simulink library "acc"  (R2021b)
settings: Solver=VariableStepAuto  StartTime=0.0  StopTime=10.0  RelTol=1e-3
undefined symbols (not defined in the file or in its folder): AACC_CondensorFanReq_X_enum, AACC_EWP1CCUReq_X_C, AACC_EWP1EDUReq_X_C, AACC_EWP1HVBReq_X_C, AACC_EWP2CCUReq_X_C, AACC_EWP2EDUReq_X_C, AACC_EWP2HVBReq_X_C, AACC_FWV1CCUReq_X_C, AACC_FWV1EDUReq_X_C, AACC_FWV1HVBReq_X_C, AACC_FWV2CCUReq_X_C, AACC_FWV2EDUReq_X_C, AACC_FWV2HVBReq_X_C, AACC_TWVCCUReq_X_C, AACC_TWVEDUReq_X_C, AACC_TWVHVBReq_X_C, ENUM_ACCMODE_CHARGING, ENUM_ACCMODE_COOLING, ENUM_ACCMODE_OFF, ENUM_ACCMODE_SERVICE, ENUM_ACREQ_COOLING, ENUM_ACREQ_NOREQUEST, ENUM_CHILLERINITREQ_NONE, ENUM_CHILLERINITREQ_START, ENUM_CHILLERINITREQ_WAITING, ENUM_CHILLERINITSTA_FINISH, ENUM_CHILLERINITSTA_INPROCESS, ENUM_COOLFANREQ_HI, ENUM_COOLFANREQ_LOW, ENUM_COOLFANREQ_OFF, ENUM_EACENDEM_SHUTDOWN, ENUM_EACENDEM_START, ENUM_EACENSTA_RUN, ENUM_EBSBRKSW_PRESSED, ENUM_EBSBRKSW_RELEASED, ENUM_EHPSENDEM_SHUTDOWN, ENUM_EHPSENDEM_START, ENUM_EPBSTARAW_SET, ENUM_GEARACTUALPOSN_N, ENUM_GEARACTUALPOSN_P, ENUM_LVBATTSTA_FAIL, ENUM_LVBATTSTA_NORMAL, ENUM_PMMMODE_CHARGE, ENUM_PMMMODE_DRIVE, ENUM_PMMMODE_LVBATCHRG, ENUM_PMMMODE_POWERUP, ENUM_POWERSTA_OFF, ENUM_POWERSTA_ON, ENUM_POWERSTA_READY, ENUM_POWERSTA_STANDBY, ENUM_PUSTATE_COMPLETED, ENUM_THCMSYS_INACTIVE, FALSE, KACC_CACEnableFailTime_s, KACC_CCUFanHighOffTemp_C, KACC_CCUFanHighOnTemp_C, KACC_CCUFanLowOffTemp_C, KACC_CCUFanLowOnTemp_C, KACC_ChillerInitTime_s, KACC_ChillerStartTime_s ... (+77)
libraries: hcu_lib x10, simulink x1
(part 2 of 2)

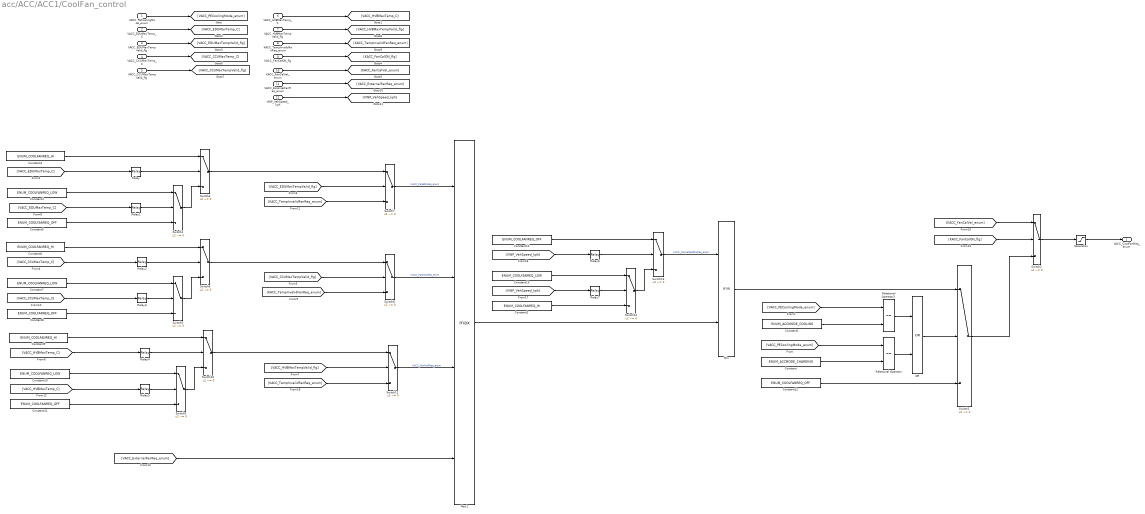
== system acc/ACC/ACC1/CoolFan_control ==
  VACC_PECoolingMode_enum : Inport
  VACC_EDUMaxTemp_C : Inport  Port=2
  VACC_EDUMaxTempValid_flg : Inport  Port=3
  VACC_CCUMaxTemp_C : Inport  Port=4
  VACC_CCUMaxTempValid_flg : Inport  Port=5
  VACC_HVBMaxTemp_C : Inport  Port=6
  VACC_HVBMaxTempValid_flg : Inport  Port=7
  KACC_TempInvalidFanReq_enum : Inport  Port=8
  KACC_FanCalON_flg : Inport  Port=9
  KACC_FanCalVal_enum : Inport  Port=10
  VACC_ExternalFanReq_enum : Inport  Port=11
  VINP_VehSpeed_kph : Inport  Port=12
  Constant : Constant  Value=ENUM_ACCMODE_CHARGING
  Constant1 : Constant  Value=ENUM_ACCMODE_COOLING
  Constant{4,7,10,13} (4 alike) : Constant  Value=ENUM_COOLFANREQ_LOW
  Constant{5,8,11..12,14} (5 alike) : Constant  Value=ENUM_COOLFANREQ_OFF
  Constant{2..3,6,9} (4 alike) : Constant  Value=ENUM_COOLFANREQ_HI
  Max1 : MinMax  Function=max  Inputs=4
  Min : MinMax  Inputs=2
  OR : Logic  Operator=OR  AllPortsSameDT=off  OutDataTypeStr=boolean
  Relational Operator : RelationalOperator  Operator===  OutDataTypeStr=boolean  RndMeth=Simplest
  Relational Operator2 : RelationalOperator  Operator===  OutDataTypeStr=boolean  RndMeth=Simplest
  Relay : Relay  OnSwitchValue=KACC_EDUFanHighOnTemp_C  OffSwitchValue=KACC_EDUFanHighOffTemp_C
      settings: AttributesFormatString=|
      | ON: %<OnSwitchValue>
      | OFF: %<OffSwitchValue>
  Relay1 : Relay  OnSwitchValue=KACC_EDUFanLowOnTemp_C  OffSwitchValue=KACC_EDUFanLowOffTemp_C
      settings: AttributesFormatString=|
      | ON: %<OnSwitchValue>
      | OFF: %<OffSwitchValue>
  Relay2 : Relay  OnSwitchValue=KACC_CCUFanHighOnTemp_C  OffSwitchValue=KACC_CCUFanHighOffTemp_C
      settings: AttributesFormatString=|
      | ON: %<OnSwitchValue>
      | OFF: %<OffSwitchValue>
  Relay3 : Relay  OnSwitchValue=KACC_CCUFanLowOnTemp_C  OffSwitchValue=KACC_CCUFanLowOffTemp_C
      settings: AttributesFormatString=|
      | ON: %<OnSwitchValue>
      | OFF: %<OffSwitchValue>
  Relay4 : Relay  OnSwitchValue=KACC_HVBFanHighOnTemp_C  OffSwitchValue=KACC_HVBFanHighOffTemp_C
      settings: AttributesFormatString=|
      | ON: %<OnSwitchValue>
      | OFF: %<OffSwitchValue>
  Relay5 : Relay  OnSwitchValue=KACC_HVBFanLowOnTemp_C  OffSwitchValue=KACC_HVBFanLowOffTemp_C
      settings: AttributesFormatString=|
      | ON: %<OnSwitchValue>
      | OFF: %<OffSwitchValue>
  Relay6 : Relay  OnSwitchValue=KACC_VehSpdFanLowOff_kph  OffSwitchValue=KACC_VehSpdFanLowOn_kph
      settings: AttributesFormatString=|
      | ON: %<OnSwitchValue>
      | OFF: %<OffSwitchValue>
  Relay7 : Relay  OnSwitchValue=KACC_VehSpdFanHighOff_kph  OffSwitchValue=KACC_VehSpdFanHighOn_kph
      settings: AttributesFormatString=|
      | ON: %<OnSwitchValue>
      | OFF: %<OffSwitchValue>
  Saturation : Saturate  UpperLimit=2  LowerLimit=0
      settings: AttributesFormatString=|
      | LowerLimi: %<LowerLimit>
      | UpperLimit: %<UpperLimit>
  Switch{1..13} (13 alike) : Switch  Criteria=u2 ~= 0
      settings: AttributesFormatString=%<Criteria>
  VACC_CoolFanReq_enum : Outport
  wires:
  Min/1 -> Switch1/1
  Switch13/1 -> Min/1  "VACC_FanVehSpdDisReq_enum"
  Max1/1 -> Min/2
  Constant2/1 -> Switch12/3
  [VINP_VehSpeed_kph] -> Relay7/1
  Constant14/1 -> Switch13/1
  [VINP_VehSpeed_kph] -> Relay6/1
  Switch12/1 -> Switch13/3
  Constant13/1 -> Switch12/1
  Relay7/1 -> Switch12/2
  Relay6/1 -> Switch13/2
  Constant12/1 -> Switch1/3
  [VACC_ExternalFanReq_enum] -> Max1/4
  Switch11/1 -> Max1/3  "VACC_FanHVBReq_enum"
  Switch8/1 -> Max1/2  "VACC_FanCCUReq_enum"
  Switch7/1 -> Max1/1  "VACC_FanEDUReq_enum"
  VINP_VehSpeed_kph/1 -> [VINP_VehSpeed_kph]
  [KACC_TempInvalidFanReq_enum] -> Switch11/3
  Switch10/1 -> Switch11/1
  Constant11/1 -> Switch9/3
  Constant10/1 -> Switch9/1
  Relay5/1 -> Switch9/2
  Switch9/1 -> Switch10/3
  Constant9/1 -> Switch10/1
  Relay4/1 -> Switch10/2
  [VACC_HVBMaxTempValid_flg] -> Switch11/2
  [VACC_HVBMaxTemp_C] -> Relay4/1
  [VACC_HVBMaxTemp_C] -> Relay5/1
  [VACC_CCUMaxTemp_C] -> Relay3/1
  [VACC_CCUMaxTemp_C] -> Relay2/1
  [VACC_CCUMaxTempValid_flg] -> Switch8/2
  Relay2/1 -> Switch6/2
  Constant6/1 -> Switch6/1
  Switch5/1 -> Switch6/3
  Relay3/1 -> Switch5/2
  Constant7/1 -> Switch5/1
  Constant8/1 -> Switch5/3
  Switch6/1 -> Switch8/1
  [KACC_TempInvalidFanReq_enum] -> Switch8/3
  [KACC_TempInvalidFanReq_enum] -> Switch7/3
  [VACC_EDUMaxTempValid_flg] -> Switch7/2
  Switch4/1 -> Switch7/1
  Constant5/1 -> Switch3/3
  Constant4/1 -> Switch3/1
  Relay1/1 -> Switch3/2
  [VACC_EDUMaxTemp_C] -> Relay1/1
  Switch3/1 -> Switch4/3
  Constant3/1 -> Switch4/1
  Relay/1 -> Switch4/2
  [VACC_EDUMaxTemp_C] -> Relay/1
  VACC_ExternalFanReq_enum/1 -> [VACC_ExternalFanReq_enum]
  [KACC_FanCalVal_enum] -> Switch2/1
  [KACC_FanCalON_flg] -> Switch2/2
  KACC_FanCalVal_enum/1 -> [KACC_FanCalVal_enum]
  KACC_FanCalON_flg/1 -> [KACC_FanCalON_flg]
  Saturation/1 -> VACC_CoolFanReq_enum/1
  Switch2/1 -> Saturation/1
  VACC_PECoolingMode_enum/1 -> [VACC_PECoolingMode_enum]
  [VACC_PECoolingMode_enum] -> Relational Operator/1
  [VACC_PECoolingMode_enum] -> Relational Operator2/1
  Constant1/1 -> Relational Operator2/2
  Constant/1 -> Relational Operator/2
  Switch1/1 -> Switch2/3
  VACC_HVBMaxTemp_C/1 -> [VACC_HVBMaxTemp_C]
  Relational Operator2/1 -> OR/1
  Relational Operator/1 -> OR/2
  OR/1 -> Switch1/2
  VACC_EDUMaxTemp_C/1 -> [VACC_EDUMaxTemp_C]
  VACC_EDUMaxTempValid_flg/1 -> [VACC_EDUMaxTempValid_flg]
  VACC_CCUMaxTemp_C/1 -> [VACC_CCUMaxTemp_C]
  VACC_CCUMaxTempValid_flg/1 -> [VACC_CCUMaxTempValid_flg]
  VACC_HVBMaxTempValid_flg/1 -> [VACC_HVBMaxTempValid_flg]
  KACC_TempInvalidFanReq_enum/1 -> [KACC_TempInvalidFanReq_enum]

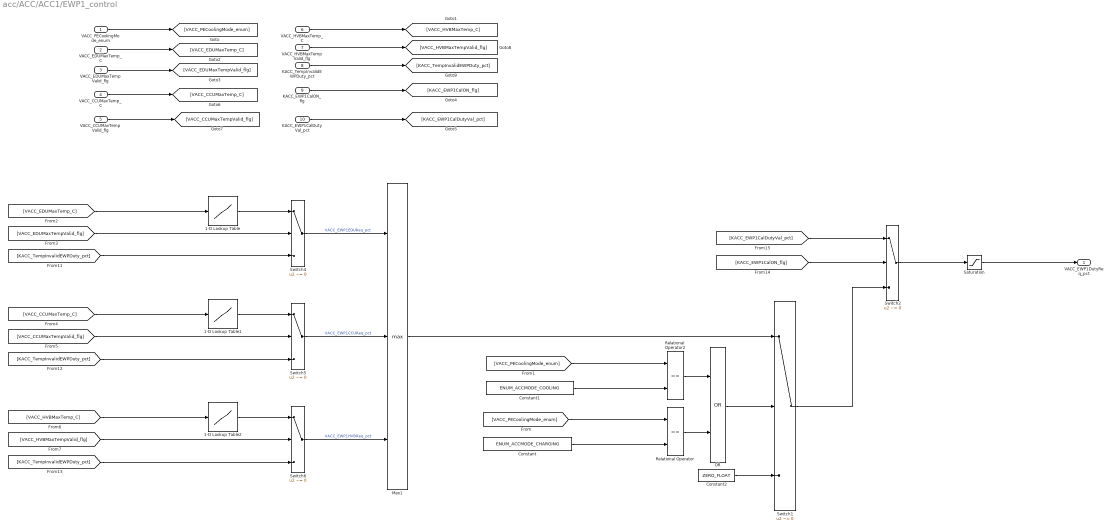
== system acc/ACC/ACC1/EWP1_control ==
  VACC_PECoolingMode_enum : Inport
  VACC_EDUMaxTemp_C : Inport  Port=2
  VACC_EDUMaxTempValid_flg : Inport  Port=3
  VACC_CCUMaxTemp_C : Inport  Port=4
  VACC_CCUMaxTempValid_flg : Inport  Port=5
  VACC_HVBMaxTemp_C : Inport  Port=6
  VACC_HVBMaxTempValid_flg : Inport  Port=7
  KACC_TempInvalidEWPDuty_pct : Inport  Port=8
  KACC_EWP1CalON_flg : Inport  Port=9
  KACC_EWP1CalDutyVal_pct : Inport  Port=10
  1-D Lookup Table : Lookup_n-D  NumberOfTableDimensions=1  BreakpointsForDimension1=AACC_EWP1EDUReq_X_C  Table=MACC_EWP1EDUReq_Y_pct  UseLastTableValue=on  InternalRulePriority=Speed  RndMeth=Simplest  InputSameDT=on
  1-D Lookup Table1 : Lookup_n-D  NumberOfTableDimensions=1  BreakpointsForDimension1=AACC_EWP1CCUReq_X_C  Table=MACC_EWP1CCUReq_Y_pct  UseLastTableValue=on  InternalRulePriority=Speed  RndMeth=Simplest  InputSameDT=on
  1-D Lookup Table2 : Lookup_n-D  NumberOfTableDimensions=1  BreakpointsForDimension1=AACC_EWP1HVBReq_X_C  Table=MACC_EWP1HVBReq_Y_pct  UseLastTableValue=on  InternalRulePriority=Speed  RndMeth=Simplest  InputSameDT=on
  Constant : Constant  Value=ENUM_ACCMODE_CHARGING
  Constant1 : Constant  Value=ENUM_ACCMODE_COOLING
  Constant2 : Constant  Value=ZERO_FLOAT
  Max1 : MinMax  Function=max  Inputs=3
  OR : Logic  Operator=OR  AllPortsSameDT=off  OutDataTypeStr=boolean
  Relational Operator : RelationalOperator  Operator===  OutDataTypeStr=boolean  RndMeth=Simplest
  Relational Operator2 : RelationalOperator  Operator===  OutDataTypeStr=boolean  RndMeth=Simplest
  Saturation : Saturate  UpperLimit=100  LowerLimit=0
      settings: AttributesFormatString=|
      | LowerLimi: %<LowerLimit>
      | UpperLimit: %<UpperLimit>
  Switch{1..2,4..6} (5 alike) : Switch  Criteria=u2 ~= 0
      settings: AttributesFormatString=%<Criteria>
  VACC_EWP1DutyReq_pct : Outport
  wires:
  Saturation/1 -> VACC_EWP1DutyReq_pct/1
  [KACC_EWP1CalDutyVal_pct] -> Switch2/1
  [KACC_EWP1CalON_flg] -> Switch2/2
  [KACC_TempInvalidEWPDuty_pct] -> Switch6/3
  [VACC_HVBMaxTemp_C] -> 1-D Lookup Table2/1
  [VACC_HVBMaxTempValid_flg] -> Switch6/2
  1-D Lookup Table2/1 -> Switch6/1
  Switch6/1 -> Max1/3  "VACC_EWP1HVBReq_pct"
  [KACC_TempInvalidEWPDuty_pct] -> Switch5/3
  [VACC_CCUMaxTempValid_flg] -> Switch5/2
  1-D Lookup Table1/1 -> Switch5/1
  [VACC_CCUMaxTemp_C] -> 1-D Lookup Table1/1
  1-D Lookup Table/1 -> Switch4/1
  [VACC_EDUMaxTemp_C] -> 1-D Lookup Table/1
  [KACC_TempInvalidEWPDuty_pct] -> Switch4/3
  [VACC_EDUMaxTempValid_flg] -> Switch4/2
  KACC_EWP1CalDutyVal_pct/1 -> [KACC_EWP1CalDutyVal_pct]
  KACC_EWP1CalON_flg/1 -> [KACC_EWP1CalON_flg]
  Switch2/1 -> Saturation/1
  VACC_PECoolingMode_enum/1 -> [VACC_PECoolingMode_enum]
  [VACC_PECoolingMode_enum] -> Relational Operator/1
  [VACC_PECoolingMode_enum] -> Relational Operator2/1
  Max1/1 -> Switch1/1
  Constant1/1 -> Relational Operator2/2
  Constant/1 -> Relational Operator/2
  Switch1/1 -> Switch2/3
  VACC_HVBMaxTemp_C/1 -> [VACC_HVBMaxTemp_C]
  Relational Operator2/1 -> OR/1
  Relational Operator/1 -> OR/2
  OR/1 -> Switch1/2
  Constant2/1 -> Switch1/3
  VACC_EDUMaxTemp_C/1 -> [VACC_EDUMaxTemp_C]
  VACC_EDUMaxTempValid_flg/1 -> [VACC_EDUMaxTempValid_flg]
  VACC_CCUMaxTemp_C/1 -> [VACC_CCUMaxTemp_C]
  VACC_CCUMaxTempValid_flg/1 -> [VACC_CCUMaxTempValid_flg]
  VACC_HVBMaxTempValid_flg/1 -> [VACC_HVBMaxTempValid_flg]
  KACC_TempInvalidEWPDuty_pct/1 -> [KACC_TempInvalidEWPDuty_pct]
  Switch4/1 -> Max1/1  "VACC_EWP1EDUReq_pct"
  Switch5/1 -> Max1/2  "VACC_EWP1CCUReq_pct"

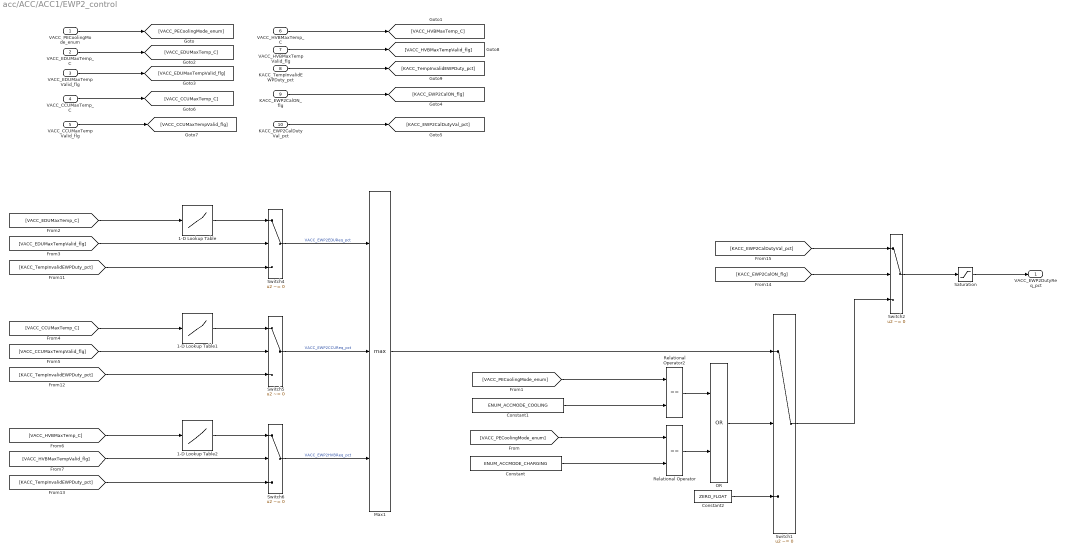
== system acc/ACC/ACC1/EWP2_control ==
  VACC_PECoolingMode_enum : Inport
  VACC_EDUMaxTemp_C : Inport  Port=2
  VACC_EDUMaxTempValid_flg : Inport  Port=3
  VACC_CCUMaxTemp_C : Inport  Port=4
  VACC_CCUMaxTempValid_flg : Inport  Port=5
  VACC_HVBMaxTemp_C : Inport  Port=6
  VACC_HVBMaxTempValid_flg : Inport  Port=7
  KACC_TempInvalidEWPDuty_pct : Inport  Port=8
  KACC_EWP2CalON_flg : Inport  Port=9
  KACC_EWP2CalDutyVal_pct : Inport  Port=10
  1-D Lookup Table : Lookup_n-D  NumberOfTableDimensions=1  BreakpointsForDimension1=AACC_EWP2EDUReq_X_C  Table=MACC_EWP2EDUReq_Y_pct  UseLastTableValue=on  InternalRulePriority=Speed  RndMeth=Simplest  InputSameDT=on
  1-D Lookup Table1 : Lookup_n-D  NumberOfTableDimensions=1  BreakpointsForDimension1=AACC_EWP2CCUReq_X_C  Table=MACC_EWP2CCUReq_Y_pct  UseLastTableValue=on  InternalRulePriority=Speed  RndMeth=Simplest  InputSameDT=on
  1-D Lookup Table2 : Lookup_n-D  NumberOfTableDimensions=1  BreakpointsForDimension1=AACC_EWP2HVBReq_X_C  Table=MACC_EWP2HVBReq_Y_pct  UseLastTableValue=on  InternalRulePriority=Speed  RndMeth=Simplest  InputSameDT=on
  Constant : Constant  Value=ENUM_ACCMODE_CHARGING
  Constant1 : Constant  Value=ENUM_ACCMODE_COOLING
  Constant2 : Constant  Value=ZERO_FLOAT
  Max1 : MinMax  Function=max  Inputs=3
  OR : Logic  Operator=OR  AllPortsSameDT=off  OutDataTypeStr=boolean
  Relational Operator : RelationalOperator  Operator===  OutDataTypeStr=boolean  RndMeth=Simplest
  Relational Operator2 : RelationalOperator  Operator===  OutDataTypeStr=boolean  RndMeth=Simplest
  Saturation : Saturate  UpperLimit=100  LowerLimit=0
      settings: AttributesFormatString=|
      | LowerLimi: %<LowerLimit>
      | UpperLimit: %<UpperLimit>
  Switch{1..2,4..6} (5 alike) : Switch  Criteria=u2 ~= 0
      settings: AttributesFormatString=%<Criteria>
  VACC_EWP2DutyReq_pct : Outport
  wires:
  Switch5/1 -> Max1/2  "VACC_EWP2CCUReq_pct"
  Switch4/1 -> Max1/1  "VACC_EWP2EDUReq_pct"
  KACC_TempInvalidEWPDuty_pct/1 -> [KACC_TempInvalidEWPDuty_pct]
  VACC_HVBMaxTempValid_flg/1 -> [VACC_HVBMaxTempValid_flg]
  VACC_CCUMaxTempValid_flg/1 -> [VACC_CCUMaxTempValid_flg]
  VACC_CCUMaxTemp_C/1 -> [VACC_CCUMaxTemp_C]
  VACC_EDUMaxTempValid_flg/1 -> [VACC_EDUMaxTempValid_flg]
  VACC_EDUMaxTemp_C/1 -> [VACC_EDUMaxTemp_C]
  Constant2/1 -> Switch1/3
  OR/1 -> Switch1/2
  Relational Operator/1 -> OR/2
  Relational Operator2/1 -> OR/1
  VACC_HVBMaxTemp_C/1 -> [VACC_HVBMaxTemp_C]
  Switch1/1 -> Switch2/3
  Constant/1 -> Relational Operator/2
  Constant1/1 -> Relational Operator2/2
  Max1/1 -> Switch1/1
  [VACC_PECoolingMode_enum] -> Relational Operator2/1
  [VACC_PECoolingMode_enum] -> Relational Operator/1
  VACC_PECoolingMode_enum/1 -> [VACC_PECoolingMode_enum]
  Switch2/1 -> Saturation/1
  Saturation/1 -> VACC_EWP2DutyReq_pct/1
  KACC_EWP2CalON_flg/1 -> [KACC_EWP2CalON_flg]
  KACC_EWP2CalDutyVal_pct/1 -> [KACC_EWP2CalDutyVal_pct]
  [VACC_EDUMaxTempValid_flg] -> Switch4/2
  [KACC_TempInvalidEWPDuty_pct] -> Switch4/3
  [VACC_EDUMaxTemp_C] -> 1-D Lookup Table/1
  1-D Lookup Table/1 -> Switch4/1
  [VACC_CCUMaxTemp_C] -> 1-D Lookup Table1/1
  1-D Lookup Table1/1 -> Switch5/1
  [VACC_CCUMaxTempValid_flg] -> Switch5/2
  [KACC_TempInvalidEWPDuty_pct] -> Switch5/3
  Switch6/1 -> Max1/3  "VACC_EWP2HVBReq_pct"
  1-D Lookup Table2/1 -> Switch6/1
  [VACC_HVBMaxTempValid_flg] -> Switch6/2
  [VACC_HVBMaxTemp_C] -> 1-D Lookup Table2/1
  [KACC_TempInvalidEWPDuty_pct] -> Switch6/3
  [KACC_EWP2CalON_flg] -> Switch2/2
  [KACC_EWP2CalDutyVal_pct] -> Switch2/1

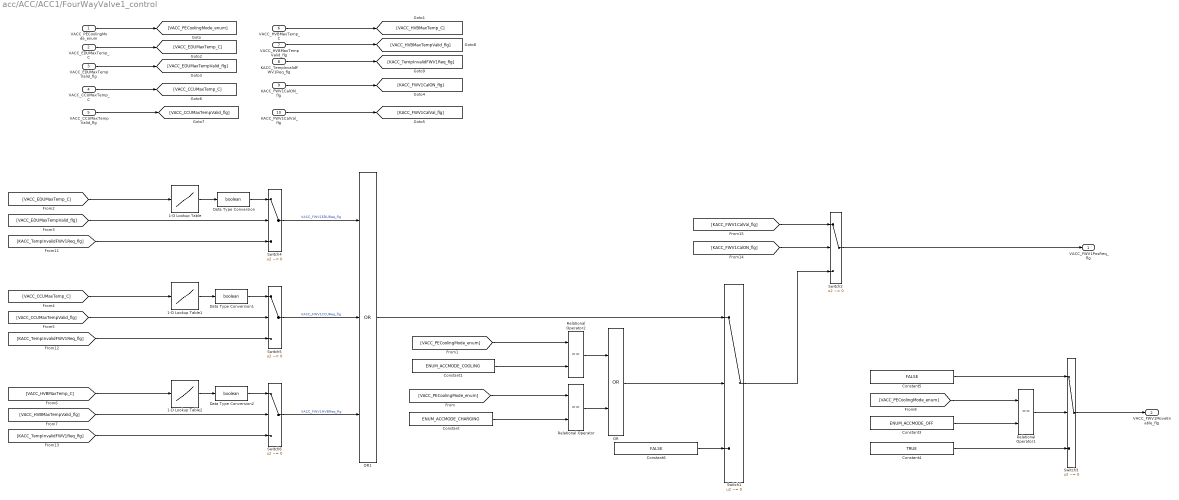
== system acc/ACC/ACC1/FourWayValve1_control ==
  VACC_PECoolingMode_enum : Inport
  VACC_EDUMaxTemp_C : Inport  Port=2
  VACC_EDUMaxTempValid_flg : Inport  Port=3
  VACC_CCUMaxTemp_C : Inport  Port=4
  VACC_CCUMaxTempValid_flg : Inport  Port=5
  VACC_HVBMaxTemp_C : Inport  Port=6
  VACC_HVBMaxTempValid_flg : Inport  Port=7
  KACC_TempInvalidFWV1Req_flg : Inport  Port=8
  KACC_FWV1CalON_flg : Inport  Port=9
  KACC_FWV1CalVal_flg : Inport  Port=10
  1-D Lookup Table : Lookup_n-D  NumberOfTableDimensions=1  BreakpointsForDimension1=AACC_FWV1EDUReq_X_C  Table=MACC_FWV1EDUReq_Y_flg  InterpMethod=Flat  UseLastTableValue=on  InternalRulePriority=Speed  RndMeth=Simplest  InputSameDT=on
  1-D Lookup Table1 : Lookup_n-D  NumberOfTableDimensions=1  BreakpointsForDimension1=AACC_FWV1CCUReq_X_C  Table=MACC_FWV1CCUReq_Y_flg  InterpMethod=Flat  UseLastTableValue=on  InternalRulePriority=Speed  RndMeth=Simplest  InputSameDT=on
  1-D Lookup Table2 : Lookup_n-D  NumberOfTableDimensions=1  BreakpointsForDimension1=AACC_FWV1HVBReq_X_C  Table=MACC_FWV1HVBReq_Y_flg  InterpMethod=Flat  UseLastTableValue=on  InternalRulePriority=Speed  RndMeth=Simplest  InputSameDT=on
  Constant : Constant  Value=ENUM_ACCMODE_CHARGING
  Constant1 : Constant  Value=ENUM_ACCMODE_COOLING
  Constant3 : Constant  Value=ENUM_ACCMODE_OFF
  Constant4 : Constant  Value=TRUE
  Constant5 : Constant  Value=FALSE
  Constant6 : Constant  Value=FALSE
  Data Type Conversion : DataTypeConversion  OutDataTypeStr=boolean
  Data Type Conversion1 : DataTypeConversion  OutDataTypeStr=boolean
  Data Type Conversion2 : DataTypeConversion  OutDataTypeStr=boolean
  OR : Logic  Operator=OR  AllPortsSameDT=off  OutDataTypeStr=boolean
  OR1 : Logic  Operator=OR  Inputs=3  AllPortsSameDT=off  OutDataTypeStr=boolean
  Relational Operator : RelationalOperator  Operator===  OutDataTypeStr=boolean  RndMeth=Simplest
  Relational Operator1 : RelationalOperator  Operator===  OutDataTypeStr=boolean  RndMeth=Simplest
  Relational Operator2 : RelationalOperator  Operator===  OutDataTypeStr=boolean  RndMeth=Simplest
  Switch{1..6} (6 alike) : Switch  Criteria=u2 ~= 0
      settings: AttributesFormatString=%<Criteria>
  VACC_FWV1PosReq_flg : Outport
  VACC_FWV1MoveEnable_flg : Outport  Port=2
  wires:
  Data Type Conversion2/1 -> Switch6/1
  Data Type Conversion1/1 -> Switch5/1
  Data Type Conversion/1 -> Switch4/1
  OR1/1 -> Switch1/1
  Constant6/1 -> Switch1/3
  [KACC_FWV1CalVal_flg] -> Switch2/1
  [KACC_FWV1CalON_flg] -> Switch2/2
  [KACC_TempInvalidFWV1Req_flg] -> Switch6/3
  [VACC_HVBMaxTemp_C] -> 1-D Lookup Table2/1
  [VACC_HVBMaxTempValid_flg] -> Switch6/2
  1-D Lookup Table2/1 -> Data Type Conversion2/1
  Switch6/1 -> OR1/3  "VACC_FWV1HVBReq_flg"
  [KACC_TempInvalidFWV1Req_flg] -> Switch5/3
  [VACC_CCUMaxTempValid_flg] -> Switch5/2
  1-D Lookup Table1/1 -> Data Type Conversion1/1
  [VACC_CCUMaxTemp_C] -> 1-D Lookup Table1/1
  1-D Lookup Table/1 -> Data Type Conversion/1
  [VACC_EDUMaxTemp_C] -> 1-D Lookup Table/1
  [KACC_TempInvalidFWV1Req_flg] -> Switch4/3
  [VACC_EDUMaxTempValid_flg] -> Switch4/2
  KACC_FWV1CalVal_flg/1 -> [KACC_FWV1CalVal_flg]
  KACC_FWV1CalON_flg/1 -> [KACC_FWV1CalON_flg]
  Switch2/1 -> VACC_FWV1PosReq_flg/1
  VACC_PECoolingMode_enum/1 -> [VACC_PECoolingMode_enum]
  [VACC_PECoolingMode_enum] -> Relational Operator/1
  [VACC_PECoolingMode_enum] -> Relational Operator2/1
  Constant1/1 -> Relational Operator2/2
  Constant/1 -> Relational Operator/2
  Switch1/1 -> Switch2/3
  VACC_HVBMaxTemp_C/1 -> [VACC_HVBMaxTemp_C]
  Relational Operator2/1 -> OR/1
  Relational Operator/1 -> OR/2
  OR/1 -> Switch1/2
  VACC_EDUMaxTemp_C/1 -> [VACC_EDUMaxTemp_C]
  VACC_EDUMaxTempValid_flg/1 -> [VACC_EDUMaxTempValid_flg]
  VACC_CCUMaxTemp_C/1 -> [VACC_CCUMaxTemp_C]
  VACC_CCUMaxTempValid_flg/1 -> [VACC_CCUMaxTempValid_flg]
  VACC_HVBMaxTempValid_flg/1 -> [VACC_HVBMaxTempValid_flg]
  KACC_TempInvalidFWV1Req_flg/1 -> [KACC_TempInvalidFWV1Req_flg]
  Switch4/1 -> OR1/1  "VACC_FWV1EDUReq_flg"
  Switch5/1 -> OR1/2  "VACC_FWV1CCUReq_flg"
  Constant3/1 -> Relational Operator1/2
  [VACC_PECoolingMode_enum] -> Relational Operator1/1
  Relational Operator1/1 -> Switch3/2
  Switch3/1 -> VACC_FWV1MoveEnable_flg/1
  Constant5/1 -> Switch3/1
  Constant4/1 -> Switch3/3

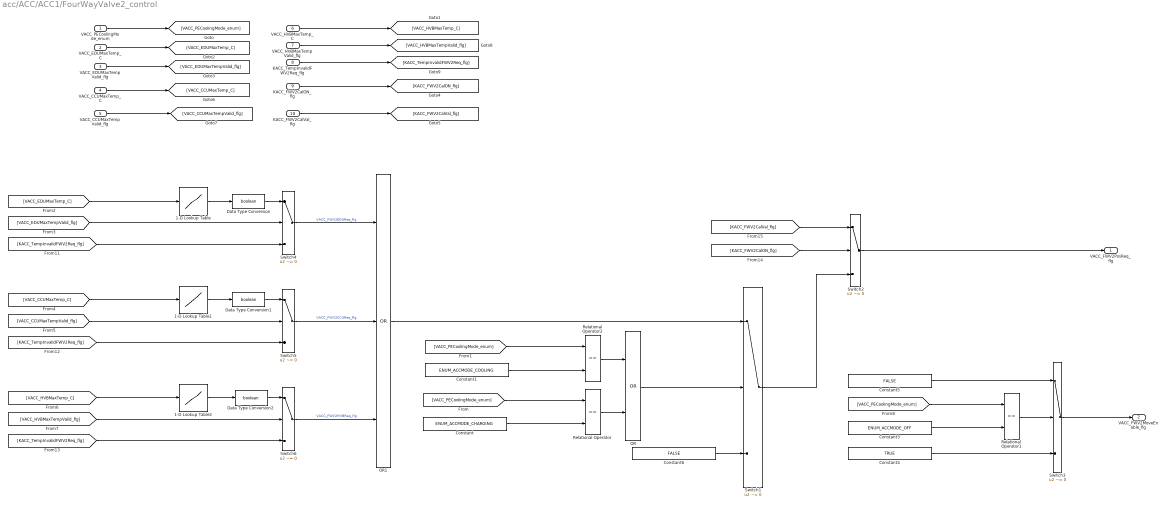
== system acc/ACC/ACC1/FourWayValve2_control ==
  VACC_PECoolingMode_enum : Inport
  VACC_EDUMaxTemp_C : Inport  Port=2
  VACC_EDUMaxTempValid_flg : Inport  Port=3
  VACC_CCUMaxTemp_C : Inport  Port=4
  VACC_CCUMaxTempValid_flg : Inport  Port=5
  VACC_HVBMaxTemp_C : Inport  Port=6
  VACC_HVBMaxTempValid_flg : Inport  Port=7
  KACC_TempInvalidFWV2Req_flg : Inport  Port=8
  KACC_FWV2CalON_flg : Inport  Port=9
  KACC_FWV2CalVal_flg : Inport  Port=10
  1-D Lookup Table : Lookup_n-D  NumberOfTableDimensions=1  BreakpointsForDimension1=AACC_FWV2EDUReq_X_C  Table=MACC_FWV2EDUReq_Y_flg  InterpMethod=Flat  UseLastTableValue=on  InternalRulePriority=Speed  RndMeth=Simplest  InputSameDT=on
  1-D Lookup Table1 : Lookup_n-D  NumberOfTableDimensions=1  BreakpointsForDimension1=AACC_FWV2CCUReq_X_C  Table=MACC_FWV2CCUReq_Y_flg  InterpMethod=Flat  UseLastTableValue=on  InternalRulePriority=Speed  RndMeth=Simplest  InputSameDT=on
  1-D Lookup Table2 : Lookup_n-D  NumberOfTableDimensions=1  BreakpointsForDimension1=AACC_FWV2HVBReq_X_C  Table=MACC_FWV2HVBReq_Y_flg  InterpMethod=Flat  UseLastTableValue=on  InternalRulePriority=Speed  RndMeth=Simplest  InputSameDT=on
  Constant : Constant  Value=ENUM_ACCMODE_CHARGING
  Constant1 : Constant  Value=ENUM_ACCMODE_COOLING
  Constant3 : Constant  Value=ENUM_ACCMODE_OFF
  Constant4 : Constant  Value=TRUE
  Constant5 : Constant  Value=FALSE
  Constant6 : Constant  Value=FALSE
  Data Type Conversion : DataTypeConversion  OutDataTypeStr=boolean
  Data Type Conversion1 : DataTypeConversion  OutDataTypeStr=boolean
  Data Type Conversion2 : DataTypeConversion  OutDataTypeStr=boolean
  OR : Logic  Operator=OR  AllPortsSameDT=off  OutDataTypeStr=boolean
  OR1 : Logic  Operator=OR  Inputs=3  AllPortsSameDT=off  OutDataTypeStr=boolean
  Relational Operator : RelationalOperator  Operator===  OutDataTypeStr=boolean  RndMeth=Simplest
  Relational Operator1 : RelationalOperator  Operator===  OutDataTypeStr=boolean  RndMeth=Simplest
  Relational Operator2 : RelationalOperator  Operator===  OutDataTypeStr=boolean  RndMeth=Simplest
  Switch{1..6} (6 alike) : Switch  Criteria=u2 ~= 0
      settings: AttributesFormatString=%<Criteria>
  VACC_FWV2PosReq_flg : Outport
  VACC_FWV2MoveEnable_flg : Outport  Port=2
  wires:
  Data Type Conversion2/1 -> Switch6/1
  Data Type Conversion1/1 -> Switch5/1
  Data Type Conversion/1 -> Switch4/1
  Constant4/1 -> Switch3/3
  Constant5/1 -> Switch3/1
  Switch3/1 -> VACC_FWV2MoveEnable_flg/1
  Relational Operator1/1 -> Switch3/2
  [VACC_PECoolingMode_enum] -> Relational Operator1/1
  Constant3/1 -> Relational Operator1/2
  Switch5/1 -> OR1/2  "VACC_FWV2CCUReq_flg"
  Switch4/1 -> OR1/1  "VACC_FWV2EDUReq_flg"
  KACC_TempInvalidFWV2Req_flg/1 -> [KACC_TempInvalidFWV2Req_flg]
  VACC_HVBMaxTempValid_flg/1 -> [VACC_HVBMaxTempValid_flg]
  VACC_CCUMaxTempValid_flg/1 -> [VACC_CCUMaxTempValid_flg]
  VACC_CCUMaxTemp_C/1 -> [VACC_CCUMaxTemp_C]
  VACC_EDUMaxTempValid_flg/1 -> [VACC_EDUMaxTempValid_flg]
  VACC_EDUMaxTemp_C/1 -> [VACC_EDUMaxTemp_C]
  OR/1 -> Switch1/2
  Relational Operator/1 -> OR/2
  Relational Operator2/1 -> OR/1
  VACC_HVBMaxTemp_C/1 -> [VACC_HVBMaxTemp_C]
  Switch1/1 -> Switch2/3
  Constant/1 -> Relational Operator/2
  Constant1/1 -> Relational Operator2/2
  [VACC_PECoolingMode_enum] -> Relational Operator2/1
  [VACC_PECoolingMode_enum] -> Relational Operator/1
  VACC_PECoolingMode_enum/1 -> [VACC_PECoolingMode_enum]
  Switch2/1 -> VACC_FWV2PosReq_flg/1
  KACC_FWV2CalON_flg/1 -> [KACC_FWV2CalON_flg]
  KACC_FWV2CalVal_flg/1 -> [KACC_FWV2CalVal_flg]
  [VACC_EDUMaxTempValid_flg] -> Switch4/2
  [KACC_TempInvalidFWV2Req_flg] -> Switch4/3
  [VACC_EDUMaxTemp_C] -> 1-D Lookup Table/1
  1-D Lookup Table/1 -> Data Type Conversion/1
  [VACC_CCUMaxTemp_C] -> 1-D Lookup Table1/1
  1-D Lookup Table1/1 -> Data Type Conversion1/1
  [VACC_CCUMaxTempValid_flg] -> Switch5/2
  [KACC_TempInvalidFWV2Req_flg] -> Switch5/3
  Switch6/1 -> OR1/3  "VACC_FWV2HVBReq_flg"
  1-D Lookup Table2/1 -> Data Type Conversion2/1
  [VACC_HVBMaxTempValid_flg] -> Switch6/2
  [VACC_HVBMaxTemp_C] -> 1-D Lookup Table2/1
  [KACC_TempInvalidFWV2Req_flg] -> Switch6/3
  [KACC_FWV2CalON_flg] -> Switch2/2
  [KACC_FWV2CalVal_flg] -> Switch2/1
  Constant6/1 -> Switch1/3
  OR1/1 -> Switch1/1

== system acc/ACC/ACC1/Signal_convert ==
  VINP_MCUTemp_C : Inport
  VINP_MCUTempValid_flg : Inport  Port=2
  VINP_TMTemp_C : Inport  Port=3
  VINP_TMTempValid_flg : Inport  Port=4
  VINP_DCDCTemp_C : Inport  Port=5
  VINP_DCDCTempValid_flg : Inport  Port=6
  VINP_OBCTemp_C : Inport  Port=7
  VINP_OBCTempValid_flg : Inport  Port=8
  VINP_HVBMTempMax_C : Inport  Port=9
  VINP_HVBMTempMaxValid_flg : Inport  Port=10
  VINP_CondensorFanReq_enum : Inport  Port=11
  1-D Lookup Table : Lookup_n-D  NumberOfTableDimensions=1  BreakpointsForDimension1=AACC_CondensorFanReq_X_enum  Table=MACC_CondensorFanReq_Y_enum  InterpMethod=Flat  InternalRulePriority=Speed  RndMeth=Simplest  InputSameDT=on
  Data Type Conversion : DataTypeConversion  OutDataTypeStr=single
  Data Type Conversion1 : DataTypeConversion  OutDataTypeStr=boolean
  Max2 : MinMax  Function=max  Inputs=2
  Max3 : MinMax  Function=max  Inputs=2
  OR2 : Logic  AllPortsSameDT=off  OutDataTypeStr=boolean
  OR3 : Logic  AllPortsSameDT=off  OutDataTypeStr=boolean
  VACC_EDUMaxTemp_C : Outport
  VACC_EDUMaxTempValid_flg : Outport  Port=2
  VACC_CCUMaxTemp_C : Outport  Port=3
  VACC_CCUMaxTempValid_flg : Outport  Port=4
  VACC_HVBMaxTemp_C : Outport  Port=5
  VACC_HVBMaxTempValid_flg : Outport  Port=6
  VACC_ExternalFanReq_enum : Outport  Port=7
  wires:
  Data Type Conversion1/1 -> VACC_HVBMaxTempValid_flg/1
  Data Type Conversion/1 -> VACC_HVBMaxTemp_C/1
  1-D Lookup Table/1 -> VACC_ExternalFanReq_enum/1
  VINP_CondensorFanReq_enum/1 -> 1-D Lookup Table/1
  VINP_HVBMTempMaxValid_flg/1 -> Data Type Conversion1/1
  VINP_HVBMTempMax_C/1 -> Data Type Conversion/1
  OR3/1 -> VACC_CCUMaxTempValid_flg/1
  Max3/1 -> VACC_CCUMaxTemp_C/1
  VINP_OBCTempValid_flg/1 -> OR3/2
  VINP_DCDCTempValid_flg/1 -> OR3/1
  VINP_DCDCTemp_C/1 -> Max3/1
  VINP_OBCTemp_C/1 -> Max3/2
  OR2/1 -> VACC_EDUMaxTempValid_flg/1
  VINP_TMTempValid_flg/1 -> OR2/2
  VINP_MCUTempValid_flg/1 -> OR2/1
  Max2/1 -> VACC_EDUMaxTemp_C/1
  VINP_TMTemp_C/1 -> Max2/2
  VINP_MCUTemp_C/1 -> Max2/1

== system acc/ACC/ACC1/Thermal_Managemant_Mode_Determination ==
  VPMM_SysPowerMode_enum : Inport
  Constant : Constant  Value=KACC_ServiceModeON_flg
  Cooling Mode : Subsystem
  PECoolingMode : Subsystem
  Service Mode : Subsystem
  Subsystem : Subsystem
  VACC_PECoolingMode_enum : Outport  VectorParamsAs1DForOutWhenUnconnected=off
  wires:
  Constant/1 -> Service Mode/1(KACC_ServiceModeON_flg)
  [VACC_CoolingMode_flg] -> PECoolingMode/3(VACC_CoolingMode_flg)
  [VACC_ChargingMode_flg] -> PECoolingMode/2(VACC_ChargingMode_flg)
  [VACC_ServiceMode_flg] -> PECoolingMode/1(VACC_ServiceMode_flg)
  [VPMM_SysPowerMode_enum] -> Subsystem/1(VPMM_SysPowerMode_enum)
  Subsystem/1(VACC_CoolingMode_flg) -> [VACC_CoolingMode_flg]
  PECoolingMode/1(VACC_PECoolingMode_enum) -> VACC_PECoolingMode_enum/1
  [VPMM_SysPowerMode_enum] -> Cooling Mode/1(VPMM_SysPowerMode_enum)
  VPMM_SysPowerMode_enum/1 -> [VPMM_SysPowerMode_enum]
  Service Mode/1(VACC_ServiceMode_flg) -> [VACC_ServiceMode_flg]
  Cooling Mode/1(VACC_ChargingMode_flg) -> [VACC_ChargingMode_flg]

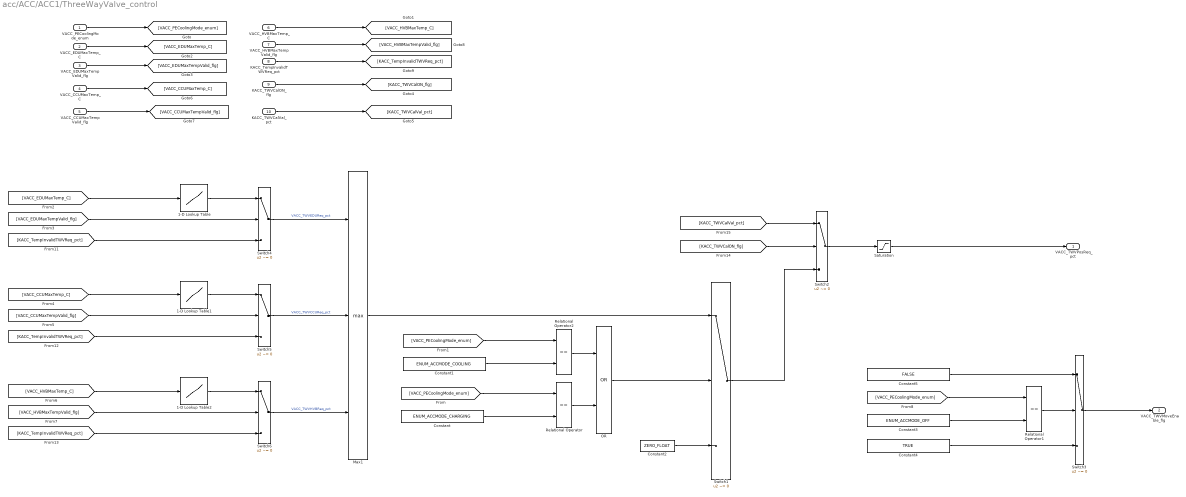
== system acc/ACC/ACC1/ThreeWayValve_control ==
  VACC_PECoolingMode_enum : Inport
  VACC_EDUMaxTemp_C : Inport  Port=2
  VACC_EDUMaxTempValid_flg : Inport  Port=3
  VACC_CCUMaxTemp_C : Inport  Port=4
  VACC_CCUMaxTempValid_flg : Inport  Port=5
  VACC_HVBMaxTemp_C : Inport  Port=6
  VACC_HVBMaxTempValid_flg : Inport  Port=7
  KACC_TempInvalidTWVReq_pct : Inport  Port=8
  KACC_TWVCalON_flg : Inport  Port=9
  KACC_TWVCalVal_pct : Inport  Port=10
  1-D Lookup Table : Lookup_n-D  NumberOfTableDimensions=1  BreakpointsForDimension1=AACC_TWVEDUReq_X_C  Table=MACC_TWVEDUReq_Y_pct  UseLastTableValue=on  InternalRulePriority=Speed  RndMeth=Simplest  InputSameDT=on
  1-D Lookup Table1 : Lookup_n-D  NumberOfTableDimensions=1  BreakpointsForDimension1=AACC_TWVCCUReq_X_C  Table=MACC_TWVCCUReq_Y_pct  UseLastTableValue=on  InternalRulePriority=Speed  RndMeth=Simplest  InputSameDT=on
  1-D Lookup Table2 : Lookup_n-D  NumberOfTableDimensions=1  BreakpointsForDimension1=AACC_TWVHVBReq_X_C  Table=MACC_TWVHVBReq_Y_pct  UseLastTableValue=on  InternalRulePriority=Speed  RndMeth=Simplest  InputSameDT=on
  Constant : Constant  Value=ENUM_ACCMODE_CHARGING
  Constant1 : Constant  Value=ENUM_ACCMODE_COOLING
  Constant2 : Constant  Value=ZERO_FLOAT
  Constant3 : Constant  Value=ENUM_ACCMODE_OFF
  Constant4 : Constant  Value=TRUE
  Constant5 : Constant  Value=FALSE
  Max1 : MinMax  Function=max  Inputs=3
  OR : Logic  Operator=OR  AllPortsSameDT=off  OutDataTypeStr=boolean
  Relational Operator : RelationalOperator  Operator===  OutDataTypeStr=boolean  RndMeth=Simplest
  Relational Operator1 : RelationalOperator  Operator===  OutDataTypeStr=boolean  RndMeth=Simplest
  Relational Operator2 : RelationalOperator  Operator===  OutDataTypeStr=boolean  RndMeth=Simplest
  Saturation : Saturate  UpperLimit=100  LowerLimit=0
      settings: AttributesFormatString=|
      | LowerLimi: %<LowerLimit>
      | UpperLimit: %<UpperLimit>
  Switch{1..6} (6 alike) : Switch  Criteria=u2 ~= 0
      settings: AttributesFormatString=%<Criteria>
  VACC_TWVPosReq_pct : Outport
  VACC_TWVMoveEnable_flg : Outport  Port=2
  wires:
  Constant4/1 -> Switch3/3
  Constant5/1 -> Switch3/1
  Switch3/1 -> VACC_TWVMoveEnable_flg/1
  Relational Operator1/1 -> Switch3/2
  [VACC_PECoolingMode_enum] -> Relational Operator1/1
  Constant3/1 -> Relational Operator1/2
  Switch5/1 -> Max1/2  "VACC_TWVCCUReq_pct"
  Switch4/1 -> Max1/1  "VACC_TWVEDUReq_pct"
  KACC_TempInvalidTWVReq_pct/1 -> [KACC_TempInvalidTWVReq_pct]
  VACC_HVBMaxTempValid_flg/1 -> [VACC_HVBMaxTempValid_flg]
  VACC_CCUMaxTempValid_flg/1 -> [VACC_CCUMaxTempValid_flg]
  VACC_CCUMaxTemp_C/1 -> [VACC_CCUMaxTemp_C]
  VACC_EDUMaxTempValid_flg/1 -> [VACC_EDUMaxTempValid_flg]
  VACC_EDUMaxTemp_C/1 -> [VACC_EDUMaxTemp_C]
  Constant2/1 -> Switch1/3
  OR/1 -> Switch1/2
  Relational Operator/1 -> OR/2
  Relational Operator2/1 -> OR/1
  VACC_HVBMaxTemp_C/1 -> [VACC_HVBMaxTemp_C]
  Switch1/1 -> Switch2/3
  Constant/1 -> Relational Operator/2
  Constant1/1 -> Relational Operator2/2
  Max1/1 -> Switch1/1
  [VACC_PECoolingMode_enum] -> Relational Operator2/1
  [VACC_PECoolingMode_enum] -> Relational Operator/1
  VACC_PECoolingMode_enum/1 -> [VACC_PECoolingMode_enum]
  Switch2/1 -> Saturation/1
  Saturation/1 -> VACC_TWVPosReq_pct/1
  KACC_TWVCalON_flg/1 -> [KACC_TWVCalON_flg]
  KACC_TWVCalVal_pct/1 -> [KACC_TWVCalVal_pct]
  [VACC_EDUMaxTempValid_flg] -> Switch4/2
  [KACC_TempInvalidTWVReq_pct] -> Switch4/3
  [VACC_EDUMaxTemp_C] -> 1-D Lookup Table/1
  1-D Lookup Table/1 -> Switch4/1
  [VACC_CCUMaxTemp_C] -> 1-D Lookup Table1/1
  1-D Lookup Table1/1 -> Switch5/1
  [VACC_CCUMaxTempValid_flg] -> Switch5/2
  [KACC_TempInvalidTWVReq_pct] -> Switch5/3
  Switch6/1 -> Max1/3  "VACC_TWVHVBReq_pct"
  1-D Lookup Table2/1 -> Switch6/1
  [VACC_HVBMaxTempValid_flg] -> Switch6/2
  [VACC_HVBMaxTemp_C] -> 1-D Lookup Table2/1
  [KACC_TempInvalidTWVReq_pct] -> Switch6/3
  [KACC_TWVCalON_flg] -> Switch2/2
  [KACC_TWVCalVal_pct] -> Switch2/1

== system acc/ACC/ACC1/Thermal_Managemant_Mode_Determination/Cooling Mode ==
  VPMM_SysPowerMode_enum : Inport
  Constant2 : Constant  Value=ENUM_PMMMODE_LVBATCHRG  SampleTime=-1
  Constant4 : Constant  Value=ENUM_PMMMODE_CHARGE  SampleTime=-1
  Logical Operator : Logic  Operator=OR  AllPortsSameDT=off  OutDataTypeStr=boolean
  Relational Operator1 : RelationalOperator  Operator===  OutDataTypeStr=boolean  RndMeth=Nearest
  Relational Operator3 : RelationalOperator  Operator===  OutDataTypeStr=boolean  RndMeth=Nearest
  VACC_ChargingMode_flg : Outport  VectorParamsAs1DForOutWhenUnconnected=off
  wires:
  [VPMM_SysPowerMode_enum] -> Relational Operator3/1
  Constant2/1 -> Relational Operator3/2
  VPMM_SysPowerMode_enum/1 -> [VPMM_SysPowerMode_enum]
  [VPMM_SysPowerMode_enum] -> Relational Operator1/1
  Constant4/1 -> Relational Operator1/2
  Relational Operator3/1 -> Logical Operator/1
  Relational Operator1/1 -> Logical Operator/2
  Logical Operator/1 -> VACC_ChargingMode_flg/1  "VACC_ChargingMode_flg"

== system acc/ACC/ACC1/Thermal_Managemant_Mode_Determination/PECoolingMode ==
  VACC_ServiceMode_flg : Inport
  VACC_ChargingMode_flg : Inport  Port=2
  VACC_CoolingMode_flg : Inport  Port=3
  Constant12 : Constant  Value=ENUM_ACCMODE_COOLING  SampleTime=-1
  Constant15 : Constant  Value=ENUM_ACCMODE_OFF  SampleTime=-1
  Constant2 : Constant  Value=ENUM_ACCMODE_CHARGING  SampleTime=-1
  Constant7 : Constant  Value=ENUM_ACCMODE_SERVICE  SampleTime=-1
  Switch1 : Switch  Criteria=u2 ~= 0
  Switch2 : Switch  Criteria=u2 ~= 0
  Switch4 : Switch  Criteria=u2 ~= 0
  VACC_PECoolingMode_enum : Outport  VectorParamsAs1DForOutWhenUnconnected=off
  wires:
  Constant15/1 -> Switch1/3
  Switch4/1 -> VACC_PECoolingMode_enum/1  "VACC_PECoolingMode_enum"
  VACC_CoolingMode_flg/1 -> Switch1/2
  Constant12/1 -> Switch1/1
  VACC_ServiceMode_flg/1 -> Switch4/2
  Constant7/1 -> Switch4/1
  Switch2/1 -> Switch4/3
  VACC_ChargingMode_flg/1 -> Switch2/2
  Switch1/1 -> Switch2/3
  Constant2/1 -> Switch2/1

== system acc/ACC/ACC1/Thermal_Managemant_Mode_Determination/Service Mode ==
  KACC_ServiceModeON_flg : Inport
  VACC_ServiceMode_flg : Outport  VectorParamsAs1DForOutWhenUnconnected=off
  wires:
  KACC_ServiceModeON_flg/1 -> VACC_ServiceMode_flg/1  "VACC_ServiceMode_flg"

== system acc/ACC/ACC1/Thermal_Managemant_Mode_Determination/Subsystem ==
  VPMM_SysPowerMode_enum : Inport
  Constant1 : Constant  Value=ENUM_PMMMODE_DRIVE  SampleTime=-1
  Constant2 : Constant  Value=ENUM_PMMMODE_POWERUP  SampleTime=-1
  Logical Operator : Logic  Operator=OR  AllPortsSameDT=off  OutDataTypeStr=boolean
  Relational Operator1 : RelationalOperator  Operator===  OutDataTypeStr=boolean  RndMeth=Nearest
  Relational Operator2 : RelationalOperator  Operator===  OutDataTypeStr=boolean  RndMeth=Nearest
  VACC_CoolingMode_flg : Outport  VectorParamsAs1DForOutWhenUnconnected=off
  wires:
  Logical Operator/1 -> VACC_CoolingMode_flg/1  "VACC_CoolingMode_flg"
  Relational Operator1/1 -> Logical Operator/2
  Relational Operator2/1 -> Logical Operator/1
  VPMM_SysPowerMode_enum/1 -> [VPMM_SysPowerMode_enum]
  [VPMM_SysPowerMode_enum] -> Relational Operator2/1
  [VPMM_SysPowerMode_enum] -> Relational Operator1/1
  Constant1/1 -> Relational Operator1/2
  Constant2/1 -> Relational Operator2/2

== stateflow chart acc/ACC/ACC/LVBattSta_Check ==
  state Check_LV_Batt
    state Check_LVBatt_Low
      en:
      VACC_ChkLVBattLowPass_flg = FALSE;
      (default) -> (junction 148) : {VACC_LVBattChkTime_s = 0;}
      (junction 148) -> (junction 149) [order 1] : [VINP_LVBattDet12V_V > KACC_LVBattErrLoThd_V]
      Check_LVBatt_Low -> (junction 148) [order 1]
      (junction 148) -> (junction 150) [order 2] : {VACC_LVBattChkTime_s += task_time_s;}
      (junction 149) -> (junction 151) : {VACC_ChkLVBattLowPass_flg = TRUE;}
      (junction 151) -> (junction 150)
    state Check_LVBatt_High
      en:
      VACC_ChkLVBattHighPass_flg = FALSE;
      (default) -> (junction 159) : {VACC_LVBattChkTime_s = 0;}
      Check_LVBatt_High -> (junction 159) [order 1]
      (junction 159) -> (junction 160) [order 1] : [VINP_LVBattDet12V_V < KACC_LVBattErrHiThd_V]
      (junction 159) -> (junction 161) [order 2] : {VACC_LVBattChkTime_s += task_time_s;}
      (junction 160) -> (junction 162) : {VACC_ChkLVBattHighPass_flg = TRUE;}
      (junction 162) -> (junction 161)
    state Check_LVBatt_Pass
      en:
      VACC_LVBattVoltSta_enum = ENUM_LVBATTSTA_NORMAL;
    state Check_LVBatt_Fail
      en:
      VACC_LVBattVoltSta_enum = ENUM_LVBATTSTA_FAIL;
    (default) -> (junction 130)
    (junction 182) -> (junction 130)
    (junction 180) -> (junction 182)
    (junction 130) -> (junction 132)
    (junction 132) -> (junction 131) [order 2]
    (junction 131) -> Check_LVBatt_Pass
    (junction 132) -> Check_LVBatt_Low [order 1] : [VPMM_LVPwrSta_flg]
    Check_LVBatt_Low -> (junction 133) [order 2] : [VACC_LVBattChkTime_s > KACC_LVBattErrFailtime_s]
    (junction 133) -> (junction 134)
    Check_LVBatt_Low -> Check_LVBatt_High [order 1] : [VACC_ChkLVBattLowPass_flg]
    Check_LVBatt_High -> (junction 134) [order 2] : [VACC_LVBattChkTime_s > KACC_LVBattErrFailtime_s]
    (junction 134) -> Check_LVBatt_Fail
    Check_LVBatt_High -> Check_LVBatt_Pass [order 1] : [VACC_ChkLVBattHighPass_flg]
    Check_LVBatt_Pass -> (junction 173)
    Check_LVBatt_Fail -> (junction 175)
    (junction 173) -> (junction 180)
    (junction 175) -> (junction 173)
  data: task_time_s input; VPMM_LVPwrSta_flg input; VINP_LVBattDet12V_V input; KACC_LVBattErrLoThd_V input; KACC_LVBattErrHiThd_V input; KACC_LVBattErrFailtime_s input; VACC_LVBattVoltSta_enum output uint8; VACC_ChkLVBattHighPass_flg local boolean; VACC_ChkLVBattLowPass_flg local boolean; VACC_LVBattChkTime_s local single; ENUM_LVBATTSTA_FAIL parameter; ENUM_LVBATTSTA_NORMAL parameter; FALSE parameter; TRUE parameter

== stateflow chart acc/ACC/ACC/EAC ==
  state EAC_Step_1
    VACC_EACPreSelfChkSta_flg = FALSE;
    state EAC_Enable
      (default) -> (junction 9) : {VACC_TimeEnSta_s = 0;
          |  VACC_EACEnDone_flg = FALSE;}
      (junction 9) -> (junction 14) [order 1] : [VINP_EACEnSta_enum == ENUM_EACENSTA_RUN]
      EAC_Enable -> (junction 9) [order 1]
      (junction 9) -> (junction 12) [order 2] : {VACC_TimeEnSta_s += task_time;}
      (junction 14) -> (junction 16) : {VACC_EACEnDone_flg = TRUE;}
      (junction 16) -> (junction 12)
    state TempStation
    (default) -> (junction 2) : {VACC_EACStep1Done_flg = FALSE;
        |  VACC_EACStep1Loop_flg = TRUE;}
    (junction 2) -> (junction 6) [order 2]
    (junction 2) -> EAC_Enable [order 1] : [VPMM_PowerSta_enum == ENUM_POWERSTA_ON]
        | {VACC_FEACEnDemand_enum = ENUM_EACENDEM_START;
        |  VACC_EACStep1Loop_flg = FALSE;}
        | %add20240718
    (junction 6) -> TempStation : {VACC_EACStep1Done_flg = FALSE;
        |  VACC_EACStep1Loop_flg = TRUE;}
    EAC_Enable -> (junction 21) [order 2] : [VACC_TimeEnSta_s > KACC_CACEnableFailTime_s]
    (junction 21) -> (junction 27) : {VACC_CACPresWarnSta_flg = TRUE;
        |  VACC_FEACEnDemand_enum = ENUM_EACENDEM_SHUTDOWN;}
    EAC_Enable -> (junction 25) [order 1] : [VACC_EACEnDone_flg]
    (junction 27) -> (junction 25)
    (junction 25) -> TempStation : {VACC_EACStep1Done_flg = TRUE;}
  state EAC_Step_2
    ex: VACC_EACPreSelfChkSta_flg = FALSE;
    (default) -> (junction 40)
    EAC_Step_2 -> (junction 40) [order 2]
    (junction 40) -> (junction 42) [order 1] : [VINP_Z24CHAAirPressureRC1Sta_kPa < 700 ||...
        |  VINP_Z24CHAAirPressureFC2Sta_kPa < 700 ||...
        |  VINP_Z24CHAAirPressurePC3Sta_kPa < 700]
    (junction 40) -> (junction 46) [order 2]
    (junction 42) -> (junction 44) : {VACC_CACPresWarnSta_flg = TRUE;}
    (junction 44) -> (junction 46)
    (junction 46) -> (junction 49)
    (junction 49) -> (junction 52) [order 1] : [VINP_Z24CHAAirPressureRC1Sta_kPa < 800 ||...
        |  VINP_Z24CHAAirPressureFC2Sta_kPa < 800]
    (junction 49) -> (junction 70) [order 2]
    (junction 52) -> (junction 150) : {VACC_FEACEnDemand_enum = ENUM_EACENDEM_START;
        |  VACC_TimeEnSta_s = 0;
        |  VACC_EACEnLoop_flg = TRUE;}
    EAC_Step_2 -> (junction 150) [order 1] : [VACC_EACEnLoop_flg]
    (junction 150) -> (junction 155) [order 2]
    (junction 155) -> (junction 73) [order 1] : [VACC_TimeEnSta_s > KACC_CACEnableFailTime_s]
    (junction 150) -> (junction 69) [order 1] : [VINP_EACEnSta_enum == ENUM_EACENSTA_RUN]
        | {VACC_EACEnLoop_flg = FALSE;}
    (junction 155) -> (junction 157) [order 2] : {VACC_TimeEnSta_s += task_time;}
    (junction 73) -> (junction 159) : {VACC_CACPresWarnSta_flg = TRUE;
        |  VACC_FEACEnDemand_enum = ENUM_EACENDEM_SHUTDOWN;
        |  VACC_EACEnLoop_flg = FALSE;}
    (junction 69) -> (junction 70)
    (junction 157) -> (junction 159)
    (junction 70) -> (junction 76)
    (junction 159) -> (junction 162)
    (junction 76) -> (junction 78) [order 1] : [VINP_Z24CHAAirPressureRC1Sta_kPa > 800 &&...
        |  VINP_Z24CHAAirPressureFC2Sta_kPa > 800]
    (junction 76) -> (junction 82) [order 2]
    (junction 78) -> (junction 80) : {VACC_EACPreSelfChkSta_flg = TRUE;}
    (junction 80) -> (junction 82)
    (junction 82) -> (junction 85)
    (junction 85) -> (junction 87) [order 1] : [VINP_Z24CHAAirPressureRC1Sta_kPa > 950 &&...
        |  VINP_Z24CHAAirPressureFC2Sta_kPa > 950]
    (junction 87) -> (junction 91) [order 1] : [VACC_TimePresEnough_s > KACC_TimePresEnoughThd_s]
    (junction 85) -> (junction 96) [order 2] : {VACC_TimePresEnough_s = 0;}
    (junction 87) -> (junction 89) [order 2] : {VACC_TimePresEnough_s += task_time;}
    (junction 91) -> (junction 93) : {VACC_CACPresWarnSta_flg = FALSE;
        |  VACC_CACTempWarnSta_flg = FALSE;
        |  VACC_FEACEnDemand_enum = ENUM_EACENDEM_SHUTDOWN;}
    (junction 89) -> (junction 93)
    (junction 93) -> (junction 113)
    (junction 96) -> (junction 98) [order 1] : [VACC_FEACEnDemand_enum == ENUM_EACENDEM_START]
    (junction 98) -> (junction 102) [order 1] : [VACC_TimeEACEnDem_s > KACC_TimeEACEnDemThd_s]
    (junction 96) -> (junction 106) [order 2] : {VACC_TimeEACEnDem_s = 0;}
    (junction 98) -> (junction 100) [order 2] : {VACC_TimeEACEnDem_s += task_time;}
    (junction 102) -> (junction 104) : {VACC_CACTempWarnSta_flg = TRUE;}
    (junction 100) -> (junction 104)
    (junction 104) -> (junction 148)
  (default) -> EAC_Step_1
  EAC_Step_1 -> EAC_Step_1 [order 2] : [VACC_EACStep1Loop_flg]
  EAC_Step_1 -> EAC_Step_2 [order 1] : [VACC_EACStep1Done_flg]
  EAC_Step_2 -> EAC_Step_1 [order 1] : [VPMM_PowerSta_enum == ENUM_POWERSTA_OFF ||...
      |  VPMM_PowerSta_enum == ENUM_POWERSTA_STANDBY]
  data: VPMM_PowerUpState_enum input; KACC_CACEnableFailTime_s parameter; KACC_TimeEACEnDemThd_s parameter; KACC_TimePresEnoughThd_s parameter; VINP_EACEnSta_enum input; VINP_Z24CHAAirPressureFC2Sta_kPa input; VINP_Z24CHAAirPressurePC3Sta_kPa input; VINP_Z24CHAAirPressureRC1Sta_kPa input; task_time input; VACC_CACPresWarnSta_flg output boolean; VACC_CACTempWarnSta_flg output boolean; VACC_EACPreSelfChkSta_flg output boolean; VACC_EACEnDone_flg local boolean; VACC_EACStep1Done_flg local boolean; VACC_FEACEnDemand_enum output uint8; VACC_TimeEACEnDem_s local single; VACC_TimeEnSta_s local single; VACC_TimePresEnough_s local single; ENUM_EACENDEM_SHUTDOWN parameter; ENUM_EACENDEM_START parameter; ENUM_EACENSTA_RUN parameter; ENUM_PUSTATE_COMPLETED parameter; FALSE parameter; TRUE parameter; VPMM_PowerSta_enum input; ENUM_POWERSTA_OFF parameter; ENUM_POWERSTA_STANDBY parameter; VACC_EACEnLoop_flg local boolean; VACC_EACStep1Loop_flg local boolean; ENUM_POWERSTA_ON parameter

== stateflow chart acc/ACC/ACC1/Chiller_control/Chiller_Initialize ==
  state MainInitialize
    en:
    VACC_ChillerInitFinish_flg = FALSE;
    VACC_ChillerInitTimeout_flg = FALSE;
    VACC_ChillerInitStart_flg = FALSE;
    VACC_ChillerInitReq_enum = ENUM_CHILLERINITREQ_NONE;
    VACC_ChillerMoveEnable_flg = FALSE;
  state ChillerInitialize
    (default) -> (junction 10) : {
        | VACC_TimeChillerInit_s = 0;
        | }
    ChillerInitialize -> (junction 10) [order 1]
    (junction 10) -> (junction 11) : {
        | VACC_ChillerInitReq_enum = ENUM_CHILLERINITREQ_START;
        | VACC_ChillerMoveEnable_flg = TRUE;
        | }
    (junction 11) -> (junction 13) [order 1] : [VINP_ChillerInitState_enum == ENUM_CHILLERINITSTA_INPROCESS]
    (junction 11) -> (junction 17) [order 2] : {
        | VACC_TimeChillerInit_s  += task_time_s;
        | }
    (junction 13) -> (junction 15) : {
        | VACC_ChillerInitStart_flg = TRUE;
        | }
    (junction 15) -> (junction 17)
  state Timeout
    en:
    VACC_ChillerInitTimeout_flg = TRUE;
    VACC_ChillerMoveEnable_flg = FALSE;
  state ChillerStart
    (default) -> (junction 28) : {
        | VACC_TimeChillerStart_s = 0;
        | }
    ChillerStart -> (junction 28) [order 1]
    (junction 28) -> (junction 29) : {
        | VACC_ChillerInitReq_enum = ENUM_CHILLERINITREQ_WAITING;
        | }
    (junction 29) -> (junction 30) [order 1] : [VINP_ChillerInitState_enum == ENUM_CHILLERINITSTA_FINISH]
    (junction 29) -> (junction 31) [order 2] : {
        | VACC_TimeChillerStart_s += task_time_s;
        | }
    (junction 30) -> (junction 32) : {
        | VACC_ChillerInitFinish_flg = TRUE;
        | VACC_ChillerInitReq_enum = ENUM_CHILLERINITREQ_NONE;
        | }
    (junction 32) -> (junction 31)
  (default) -> MainInitialize
  MainInitialize -> ChillerInitialize : [VACC_PECoolingMode_enum == ENUM_ACCMODE_COOLING ||...
      | VACC_PECoolingMode_enum == ENUM_ACCMODE_CHARGING]
  ChillerInitialize -> Timeout [order 2] : [VACC_TimeChillerInit_s > KACC_ChillerInitTime_s]
  ChillerInitialize -> ChillerStart [order 1] : [VACC_ChillerInitStart_flg]
  ChillerStart -> Timeout [order 1] : [VACC_TimeChillerStart_s > KACC_ChillerStartTime_s]
  data: KACC_ChillerInitTime_s input; KACC_ChillerStartTime_s input; VACC_PECoolingMode_enum input; VINP_ChillerInitState_enum input; task_time_s input; VACC_ChillerInitFinish_flg output; VACC_ChillerInitReq_enum output; VACC_ChillerInitTimeout_flg output; VACC_ChillerInitStart_flg local boolean; VACC_TimeChillerInit_s local single; ENUM_ACCMODE_CHARGING parameter; ENUM_ACCMODE_COOLING parameter; ENUM_CHILLERINITREQ_NONE parameter; ENUM_CHILLERINITREQ_START parameter; ENUM_CHILLERINITSTA_FINISH parameter; ENUM_CHILLERINITSTA_INPROCESS parameter; FALSE parameter; TRUE parameter; VACC_TimeChillerStart_s local single; ENUM_CHILLERINITREQ_WAITING parameter; VACC_ChillerMoveEnable_flg output boolean
